simulink model "P_ajsmt"  (R2022b)
settings: Solver=VariableStepAuto  StartTime=0.0  StopTime=3500  RelTol=1e-3
settings Model: Creator=Crapon  LastModifiedBy=Crapon

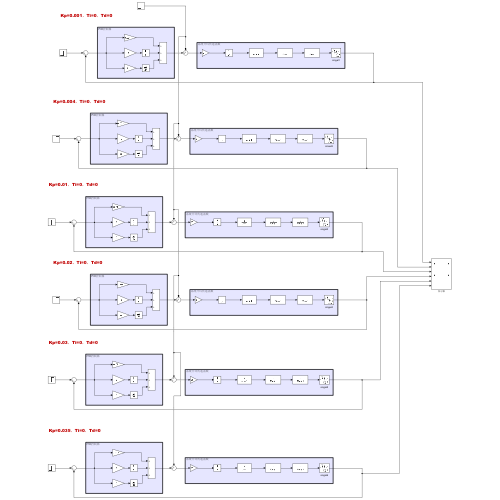
[thumbnail: Simulink's stored preview of the top-level diagram]
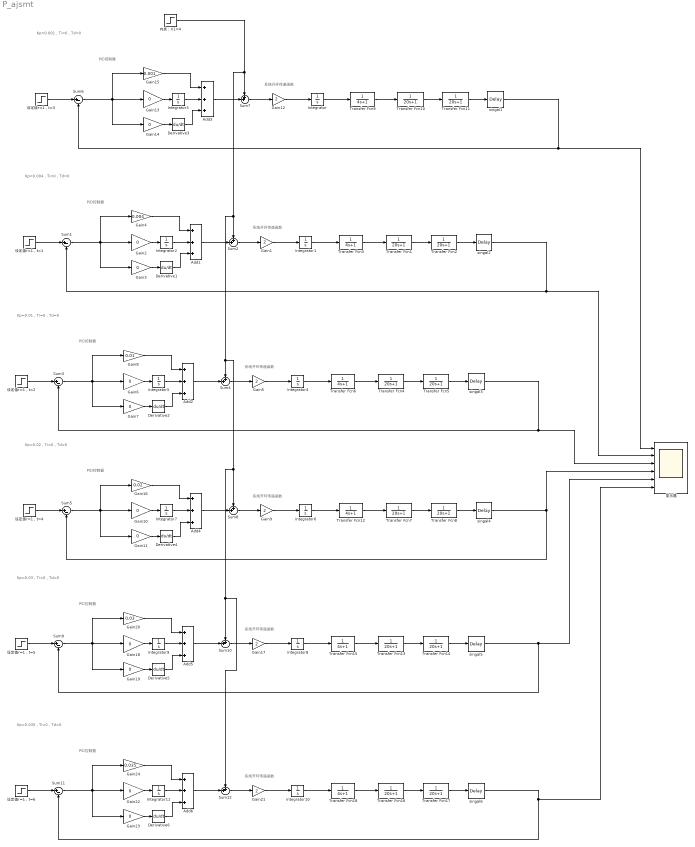
== system P_ajsmt ==
  note: PID控制器
  note: Kp=0.001，Ti=0，Td=0
  note: 系统开环传递函数
  note: PID控制器
  note: Kp=0.004，Ti=0，Td=0
  note: 系统开环传递函数
  note: Kp=0.01，Ti=0，Td=0
  note: PID控制器
  note: 系统开环传递函数
  note: Kp=0.02，Ti=0，Td=0
  note: PID控制器
  note: 系统开环传递函数
  note: Kp=0.03，Ti=0，Td=0
  note: PID控制器
  note: 系统开环传递函数
  note: Kp=0.035，Ti=0，Td=0
  note: PID控制器
  note: 系统开环传递函数
  Add{1..6} (6 alike) : Sum  Inputs=+++
  Derivative{1..6} (6 alike) : Derivative
  Gain{1,5,9,12,17,21} (6 alike) : Gain  Gain=2
  Gain{2..3,6..7,10..11,13..14,18..19,22..23} (12 alike) : Gain  Gain=0
  Gain15 : Gain  Gain=0.001
  Gain16 : Gain  Gain=0.02
  Gain20 : Gain  Gain=0.03
  Gain24 : Gain  Gain=0.035
  Gain4 : Gain  Gain=0.004
  Gain8 : Gain  Gain=0.01
  Integrator{,1..11} (12 alike) : Integrator
  Sum{1,3,5..6,9,11} (6 alike) : Sum  Inputs=|+-
  Sum{2,4,7..8,10,12} (6 alike) : Sum  Inputs=++|
  Transfer Fcn{1..2,4..5,7..8,10..11,13..14,16..17} (12 alike) : TransferFcn  Denominator=[20 1]
  Transfer Fcn{3,6,9,12,15,18} (6 alike) : TransferFcn  Denominator=[4 1]
  singal{1..6} (6 alike) : TransportDelay  DelayTime=0
  内扰：X1=4 : Step  Time=400  SampleTime=0
  显示器 : Scope  NumInputPorts=6
  设定值r=1，t={1..6} (6 alike) : Step  SampleTime=0
  wires:
  Sum7/1 -> Gain12/1
  内扰：X1=4/1 -> Sum12/1, Sum10/1, Sum8/1, Sum4/1, Sum2/1, Sum7/1
  Transfer Fcn10/1 -> Transfer Fcn11/1
  Transfer Fcn11/1 -> singal1/1
  Sum6/1 -> Gain14/1, Gain15/1, Gain13/1
  Derivative3/1 -> Add3/3
  Gain15/1 -> Add3/1
  Transfer Fcn9/1 -> Transfer Fcn10/1
  Integrator3/1 -> Add3/2
  设定值r=1，t=3/1 -> Sum6/1
  Add3/1 -> Sum7/2
  Gain13/1 -> Integrator3/1
  Gain14/1 -> Derivative3/1
  Gain12/1 -> Integrator/1
  Integrator/1 -> Transfer Fcn9/1
  singal1/1 -> Sum6/2, 显示器/1
  Gain1/1 -> Integrator1/1
  Add1/1 -> Sum2/2
  Gain3/1 -> Derivative1/1
  Gain2/1 -> Integrator2/1
  Integrator2/1 -> Add1/2
  Sum1/1 -> Gain3/1, Gain4/1, Gain2/1
  Gain4/1 -> Add1/1
  设定值r=1，t=1/1 -> Sum1/1
  Transfer Fcn1/1 -> Transfer Fcn2/1
  Derivative1/1 -> Add1/3
  Sum2/1 -> Gain1/1
  singal2/1 -> 显示器/2, Sum1/2
  Transfer Fcn3/1 -> Transfer Fcn1/1
  Transfer Fcn2/1 -> singal2/1
  Integrator1/1 -> Transfer Fcn3/1
  Transfer Fcn6/1 -> Transfer Fcn4/1
  Integrator4/1 -> Transfer Fcn6/1
  singal3/1 -> 显示器/3, Sum3/2
  Transfer Fcn5/1 -> singal3/1
  Sum3/1 -> Gain7/1, Gain8/1, Gain6/1
  Sum4/1 -> Gain5/1
  Transfer Fcn4/1 -> Transfer Fcn5/1
  设定值r=1，t=2/1 -> Sum3/1
  Derivative2/1 -> Add2/3
  Gain7/1 -> Derivative2/1
  Integrator5/1 -> Add2/2
  Gain6/1 -> Integrator5/1
  Add2/1 -> Sum4/2
  Gain5/1 -> Integrator4/1
  Gain8/1 -> Add2/1
  Transfer Fcn12/1 -> Transfer Fcn7/1
  Integrator6/1 -> Transfer Fcn12/1
  singal4/1 -> Sum5/2, 显示器/4
  Transfer Fcn8/1 -> singal4/1
  Sum5/1 -> Gain11/1, Gain16/1, Gain10/1
  Sum8/1 -> Gain9/1
  Transfer Fcn7/1 -> Transfer Fcn8/1
  设定值r=1，t=4/1 -> Sum5/1
  Derivative4/1 -> Add4/3
  Gain11/1 -> Derivative4/1
  Integrator7/1 -> Add4/2
  Gain10/1 -> Integrator7/1
  Add4/1 -> Sum8/2
  Gain9/1 -> Integrator6/1
  Gain16/1 -> Add4/1
  Transfer Fcn15/1 -> Transfer Fcn13/1
  Integrator8/1 -> Transfer Fcn15/1
  singal5/1 -> Sum9/2, 显示器/5
  Transfer Fcn14/1 -> singal5/1
  Sum9/1 -> Gain19/1, Gain20/1, Gain18/1
  Sum10/1 -> Gain17/1
  Transfer Fcn13/1 -> Transfer Fcn14/1
  设定值r=1，t=5/1 -> Sum9/1
  Derivative5/1 -> Add5/3
  Gain19/1 -> Derivative5/1
  Integrator9/1 -> Add5/2
  Gain18/1 -> Integrator9/1
  Add5/1 -> Sum10/2
  Gain17/1 -> Integrator8/1
  Gain20/1 -> Add5/1
  Transfer Fcn18/1 -> Transfer Fcn16/1
  Integrator10/1 -> Transfer Fcn18/1
  singal6/1 -> 显示器/6, Sum11/2
  Transfer Fcn17/1 -> singal6/1
  Sum11/1 -> Gain23/1, Gain24/1, Gain22/1
  Sum12/1 -> Gain21/1
  Transfer Fcn16/1 -> Transfer Fcn17/1
  设定值r=1，t=6/1 -> Sum11/1
  Derivative6/1 -> Add6/3
  Gain23/1 -> Derivative6/1
  Integrator11/1 -> Add6/2
  Gain22/1 -> Integrator11/1
  Add6/1 -> Sum12/2
  Gain21/1 -> Integrator10/1
  Gain24/1 -> Add6/1
